simulink model "example_CollectorUnglazedCONF"  (R2016b)
settings: Solver=ode45  StartTime=0.0  StopTime=24*3600  MaxStep=1800  RelTol=1e-3  EnableMultiTasking=on
libraries: carnot x13
settings Model: DataDictionary=example_collectorUnglazedSLDD.sldd  Creator=drhf  LastModifiedBy=drhf
settings DataIOCC: LimitDataPoints=on  SaveFormat=Array
settings OptimizationCC: ExpressionDepthLimit=2147483647  LifeSpan=inf
settings DebuggingCC: UnderspecifiedInitializationDetection=Classic  MergeDetectMultiDrivingBlocksExec=none  SolverPrmCheckMsg=warning  StateNameClashWarn=warning  SFUnexpectedBacktrackingDiag=warning  SFNoUnconditionalDefaultTransitionDiag=warning  SFExecutionAtInitializationDiag=none
settings HardwareCC: ProdBitPerPointer=32  ProdBitPerSizeT=32  ProdBitPerPtrDiffT=32  ProdLargestAtomicFloat=None  ProdIntDivRoundTo=Undefined  ProdEndianess=Unspecified  ProdWordSize=32  ProdHWDeviceType=32-bit Generic
settings ModelReferenceCC: PropagateSignalLabelsOutOfModel=off
settings GRTTargetCC: TargetLangStandard=C89/C90 (ANSI)  GeneratePreprocessorConditionals=Disable all  CombineOutputUpdateFcns=off  GRTInterface=on
settings ConfigComp: CovMetricSettings=dw  CovHtmlReporting=on  CovSaveCumulativeToWorkspaceVar=on  CovSaveSingleToWorkspaceVar=on  CovExternalEMLEnable=off

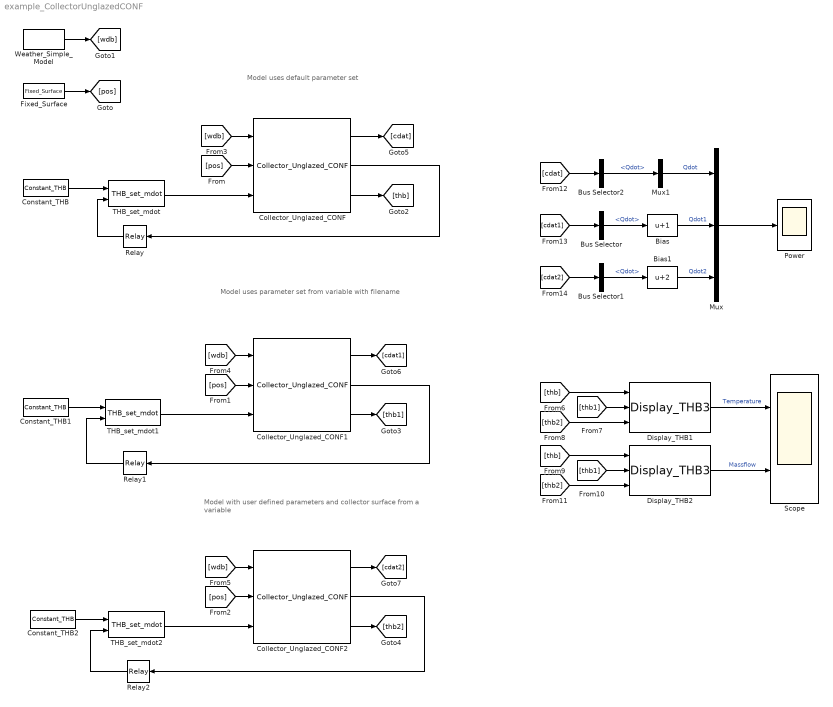
== system example_CollectorUnglazedCONF ==
  note: Model uses
      | default parameter set
  note: Model uses parameter
      | set from variable with filename
  note: Model with user defined parameters
      | and collector surface from a variable
  Bias : Bias  Bias=1
  Bias1 : Bias  Bias=2
  Bus Selector : BusSelector  OutputSignals=Qdot
  Bus Selector1 : BusSelector  OutputSignals=Qdot
  Bus Selector2 : BusSelector  OutputSignals=Qdot
  Collector_Unglazed_CONF : carnot/Source/Solar_Thermal/Collector_Unglazed_CONF  PathName='C:\repos\carnot_svn\trunk\public\library_simulink\Source\Solar_Thermal\Collector_Unglazed_CONF\parameter_set\'  FileName='DefaultCollectorUnglazed.mat'  userPath=off  tini=22  Ncollector=1  userParam=off  acol=2.5  len=2.3  fta=0.75  eps=0.9  u0c=10  u1c=3  u0l=4  u1l=3  u0g=4  u1g=1.5  u1e=0.01  hi=100  capa=7000  capf=2000  dplin=10  dpqua=10  nodes=5  SensorTimeConstant=10
  Collector_Unglazed_CONF1 : carnot/Source/Solar_Thermal/Collector_Unglazed_CONF  PathName='C:\repos\carnot_svn\trunk\public\library_simulink\Source\Solar_Thermal\Collector_Unglazed_CONF\parameter_set\'  FileName=collectorfilename  userPath=on  tini=22  Ncollector=1  userParam=off  acol=2.5  len=2.3  fta=0.75  eps=0.9  u0c=10  u1c=3  u0l=4  u1l=3  u0g=4  u1g=1.5  u1e=0.01  hi=100  capa=7000  capf=2000  dplin=10  dpqua=10  nodes=5  SensorTimeConstant=10
  Collector_Unglazed_CONF2 : carnot/Source/Solar_Thermal/Collector_Unglazed_CONF  PathName='C:\repos\carnot_svn\trunk\public\library_simulink\Source\Solar_Thermal\Collector_Unglazed_CONF\parameter_set\'  FileName='<user defined>'  userPath=off  tini=22  Ncollector=1  userParam=on  acol=collectorsurface  len=2.3  fta=0.75  eps=0.9  u0c=10  u1c=3  u0l=4  u1l=3  u0g=4  u1g=1.5  u1e=0.01  hi=100  capa=7000  capf=2000  dplin=10  dpqua=10  nodes=5  SensorTimeConstant=10
  Constant_THB : carnot/Source/Simple/Constant_THB  t=40  mdot=100/3600  p=1e5  mID=No Pressure Drop  fluid=Water  mix=0  mix2=0  mix3=0  dia=0.02  hgt=0
  Constant_THB1 : carnot/Source/Simple/Constant_THB  t=40  mdot=100/3600  p=1e5  mID=No Pressure Drop  fluid=Water  mix=0  mix2=0  mix3=0  dia=0.02  hgt=0
  Constant_THB2 : carnot/Source/Simple/Constant_THB  t=40  mdot=100/3600  p=1e5  mID=No Pressure Drop  fluid=Water  mix=0  mix2=0  mix3=0  dia=0.02  hgt=0
  Display_THB1 : carnot/Outputs/Display_THB3  t=on  m=off  p=off  id=off  mix=off  d=off
  Display_THB2 : carnot/Outputs/Display_THB3  t=off  m=on  p=off  id=off  mix=off  d=off
  Fixed_Surface : carnot/Weather/Fixed_Surface  colangle=30  colazi=0  colrot=0
  Mux : Mux  Inputs=3
  Mux1 : Mux  Inputs=1
  Power : Scope
  Relay : Relay  OnSwitchValue=47  OffSwitchValue=42  OnOutputValue=50/3600
  Relay1 : Relay  OnSwitchValue=47  OffSwitchValue=42  OnOutputValue=50/3600
  Relay2 : Relay  OnSwitchValue=47  OffSwitchValue=42  OnOutputValue=50/3600
  Scope : Scope  NumInputPorts=2
  THB_set_mdot : carnot/Source/Simple/THB_set_mdot
  THB_set_mdot1 : carnot/Source/Simple/THB_set_mdot
  THB_set_mdot2 : carnot/Source/Simple/THB_set_mdot
  Weather_Simple_Model : carnot/Weather/Weather_Simple_Model  lat=60  Ibn=900  Idg=100  tamb=5  deltaTsky=-6  rh=50  precip="10e-3/24/3600           % 10 mm in 24 h"  cloud=0.125  p=1013e2  vw=1  wdir=270
  wires:
  THB_set_mdot1/1 -> Collector_Unglazed_CONF1/3
  Display_THB1/1 -> Scope/1  "Temperature"
  Bus Selector/1 -> Bias/1  "<Qdot>"
  Bus Selector1/1 -> Bias1/1  "<Qdot>"
  Mux/1 -> Power/1
  THB_set_mdot2/1 -> Collector_Unglazed_CONF2/3
  Collector_Unglazed_CONF1/2 -> Relay1/1
  Relay1/1 -> THB_set_mdot1/2
  Relay2/1 -> THB_set_mdot2/2
  Display_THB2/1 -> Scope/2  "Massflow"
  Collector_Unglazed_CONF2/2 -> Relay2/1
  Bias/1 -> Mux/2  "Qdot1"
  Constant_THB/1 -> THB_set_mdot/1
  THB_set_mdot/1 -> Collector_Unglazed_CONF/3
  Constant_THB1/1 -> THB_set_mdot1/1
  Fixed_Surface/1 -> [pos]
  [pos] -> Collector_Unglazed_CONF/2
  [pos] -> Collector_Unglazed_CONF1/2
  [pos] -> Collector_Unglazed_CONF2/2
  [wdb] -> Collector_Unglazed_CONF/1
  [wdb] -> Collector_Unglazed_CONF1/1
  [wdb] -> Collector_Unglazed_CONF2/1
  Relay/1 -> THB_set_mdot/2
  Collector_Unglazed_CONF/2 -> Relay/1
  Weather_Simple_Model/1 -> [wdb]
  Constant_THB2/1 -> THB_set_mdot2/1
  Bus Selector2/1 -> Mux1/1  "<Qdot>"
  Collector_Unglazed_CONF/3 -> [thb]
  Collector_Unglazed_CONF1/3 -> [thb1]
  Collector_Unglazed_CONF2/3 -> [thb2]
  [thb] -> Display_THB1/1
  [thb1] -> Display_THB1/2
  [thb2] -> Display_THB1/3
  [thb] -> Display_THB2/1
  [thb1] -> Display_THB2/2
  [thb2] -> Display_THB2/3
  Mux1/1 -> Mux/1  "Qdot"
  Bias1/1 -> Mux/3  "Qdot2"
  Collector_Unglazed_CONF/1 -> [cdat]
  [cdat] -> Bus Selector2/1
  Collector_Unglazed_CONF1/1 -> [cdat1]
  [cdat1] -> Bus Selector/1
  Collector_Unglazed_CONF2/1 -> [cdat2]
  [cdat2] -> Bus Selector1/1
